simulink model "FOCCONTROL"  (R2022a)
settings: Solver=ode1  StartTime=0.0  StopTime=10  FixedStep=1e-5  RelTol=1e-5  AbsTol=1e-5
values from neighbouring files (symbols this model uses):
  A = [0 -Lq  ; Ld 0 ]    [PMSMParameters.m]
  C0 = 3.53*10.^-1    (= 0.353)    [PMSMParameters.m]
  F = 1.57*10.^-3    (= 0.00157)    [PMSMParameters.m]
  J = 5.21*10.^-3    (= 0.00521)    [PMSMParameters.m]
  Kid = Ld*((wne).^2)/Kpd    [PMSMParameters.m]
  Kim = J*((wnm).^2)/Kpm    [PMSMParameters.m]
  Kiq = Lq*((wne).^2)/Kpq    [PMSMParameters.m]
  Kpd = 2*wne*Ld*ceff-Rs    (= 1472.1)    [PMSMParameters.m]
  Kpm = 2*wnm*J*ceff-F    (= 0.25893)    [PMSMParameters.m]
  Kpq = 2*wne*Lq*ceff-Rs    (= 1122.1)    [PMSMParameters.m]
  L = [Ld 0 ; 0 Lq ]    [PMSMParameters.m]
  Ld = 0.3    [PMSMParameters.m]
  Lq = 0.23    [PMSMParameters.m]
  P = 2    [PMSMParameters.m]
  pf = 1.12    [PMSMParameters.m]
  phif = [0 ; pf]    [PMSMParameters.m]
  R = [Rs 0; 0 Rs ]    [PMSMParameters.m]
  Td = 1/fd    (= 0.001)    [PMSMParameters.m]
  VDC = 600    [PMSMParameters.m]
  VP = VDC    (= 600)    [PMSMParameters.m]
libraries: simulink x1
settings Model: Creator=ZinouAb  LastModifiedBy=ZinouAb
settings ModelReferenceCC: EnableRefExpFcnMdlSchedulingChecks=off
settings RTWCC: Description=Generic Real-Time Target

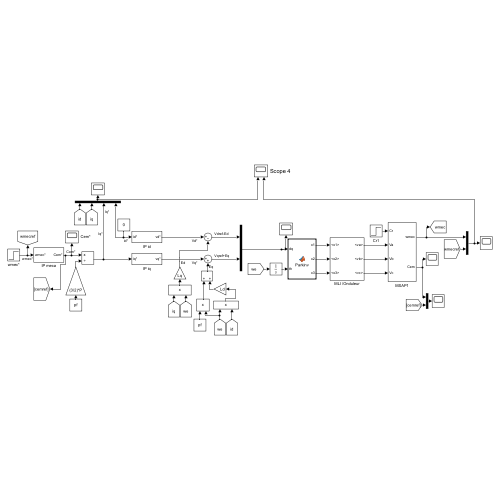
[thumbnail: Simulink's stored preview of the top-level diagram]
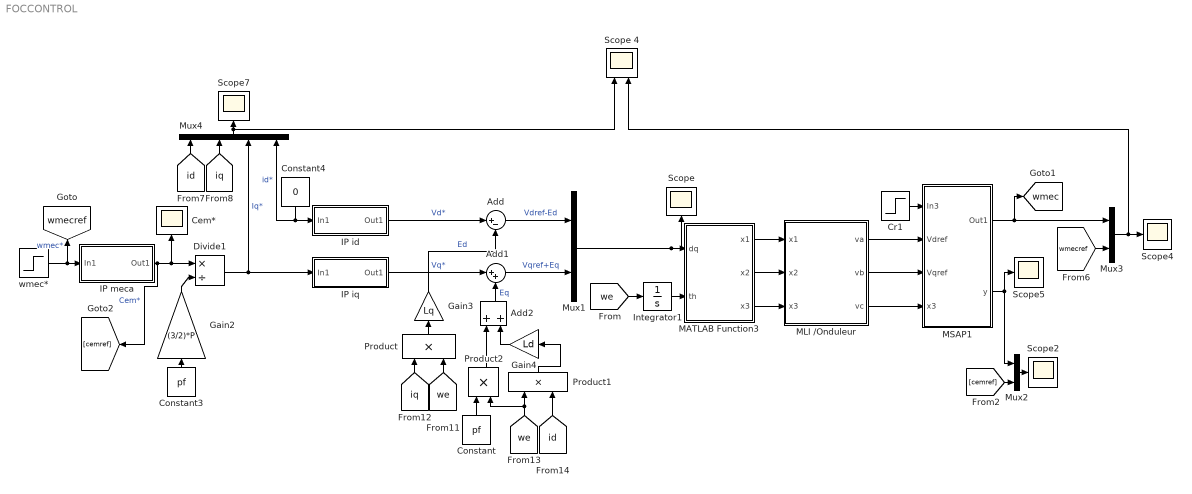
== system FOCCONTROL ==
  Add : Sum  Inputs=|+-
  Add1 : Sum  Inputs=|++
  Add2 : Sum
  Cem* : Scope
  Constant : Constant  Value=pf
  Constant3 : Constant  Value=pf
  Constant4 : Constant  Value=0
  Cr1 : Step  Time=6  After=1.9+C0  SampleTime=0
  Divide1 : Product  Inputs=*/
  Gain2 : Gain  Gain=(3/2)*P
  Gain3 : Gain  Gain=Lq
  Gain4 : Gain  Gain=Ld
  IP id : Subsystem
  IP iq : Subsystem
  IP meca : Subsystem
  Integrator1 : Integrator
  MATLAB Function3 : MATLAB Function  TreatAsAtomicUnit=on
  MLI /Onduleur : Subsystem
  MSAP1 : Subsystem
  Mux1 : Mux  Inputs=2
  Mux2 : Mux  Inputs=2
  Mux3 : Mux  Inputs=2
  Mux4 : Mux
  Product : Product
  Product1 : Product
  Product2 : Product
  Scope{,2,4..5,7} (5 alike) : Scope
  Scope 4 : Scope  NumInputPorts=2
  wmec* : Step  Time=4  After=157  SampleTime=0
  tag scope: wmec=global, wmecref=global
  wires:
  [we] -> Product/2
  MSAP1/2(y) -> Scope5/1, Mux2/1
  Gain4/1 -> Add2/2
  Constant/1 -> Product2/1
  [we] -> Product2/2, Product1/1
  Product2/1 -> Add2/1
  Product/1 -> Gain3/1
  IP iq/1(Out1) -> Add1/1  "Vq*"
  Add2/1 -> Add1/2  "Eq"
  Gain3/1 -> Add/2  "Ed"
  Product1/1 -> Gain4/1
  [id] -> Product1/2
  [iq] -> Product/1
  Constant3/1 -> Gain2/1
  Mux3/1 -> Scope 4/2, Scope4/1
  IP id/1(Out1) -> Add/1  "Vd*"
  Constant4/1 -> IP id/1(In1), Mux4/4  "id*"
  [wmecref] -> Mux3/2
  [id] -> Mux4/1
  Divide1/1 -> IP iq/1(In1), Mux4/3  "Iq*"
  wmec*/1 -> IP meca/1(In1), [wmecref]  "wmec*"
  IP meca/1(Out1) -> Divide1/1, Cem*/1, [cemref]  "Cem*"
  [iq] -> Mux4/2
  Gain2/1 -> Divide1/2
  Cr1/1 -> MSAP1/1(In3)
  Add1/1 -> Mux1/2  "Vqref+Eq"
  Integrator1/1 -> MATLAB Function3/2(th)
  Add/1 -> Mux1/1  "Vdref-Ed"
  [we] -> Integrator1/1
  Mux1/1 -> Scope/1, MATLAB Function3/1(dq)
  MLI /Onduleur/2(vb) -> MSAP1/3(Vqref)
  MLI /Onduleur/1(va) -> MSAP1/2(Vdref)
  MLI /Onduleur/3(vc) -> MSAP1/4(x3)
  MATLAB Function3/1(x1) -> MLI /Onduleur/1(x1)
  MATLAB Function3/2(x2) -> MLI /Onduleur/2(x2)
  MATLAB Function3/3(x3) -> MLI /Onduleur/3(x3)
  [cemref] -> Mux2/2
  Mux2/1 -> Scope2/1
  MSAP1/1(Out1) -> [wmec], Mux3/1
  Mux4/1 -> Scope 4/1, Scope7/1

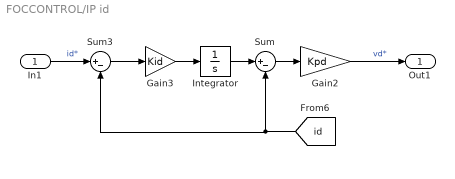
== system FOCCONTROL/IP id ==
  In1 : Inport
  Gain2 : Gain  Gain=Kpd
  Gain3 : Gain  Gain=Kid
  Integrator : Integrator
  Sum : Sum  Inputs=|+-
  Sum3 : Sum  Inputs=|+-
  Out1 : Outport
  wires:
  Integrator/1 -> Sum/1
  [id] -> Sum3/2, Sum/2
  Sum/1 -> Gain2/1
  Gain2/1 -> Out1/1  "vd*"
  Gain3/1 -> Integrator/1
  Sum3/1 -> Gain3/1
  In1/1 -> Sum3/1  "id*"

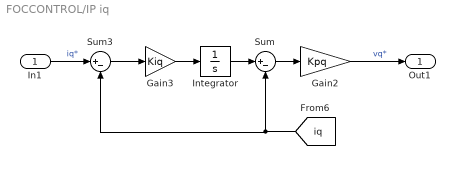
== system FOCCONTROL/IP iq ==
  In1 : Inport
  Gain2 : Gain  Gain=Kpq
  Gain3 : Gain  Gain=Kiq
  Integrator : Integrator
  Sum : Sum  Inputs=|+-
  Sum3 : Sum  Inputs=|+-
  Out1 : Outport
  wires:
  Integrator/1 -> Sum/1
  [iq] -> Sum3/2, Sum/2
  Sum/1 -> Gain2/1
  Gain2/1 -> Out1/1  "vq*"
  Gain3/1 -> Integrator/1
  Sum3/1 -> Gain3/1
  In1/1 -> Sum3/1  "iq*"

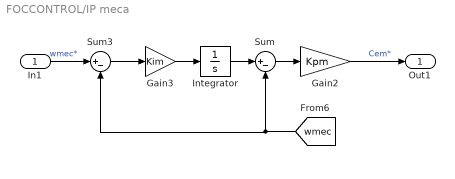
== system FOCCONTROL/IP meca ==
  In1 : Inport
  Gain2 : Gain  Gain=Kpm
  Gain3 : Gain  Gain=Kim
  Integrator : Integrator
  Sum : Sum  Inputs=|+-
  Sum3 : Sum  Inputs=|+-
  Out1 : Outport
  wires:
  Integrator/1 -> Sum/1
  [wmec] -> Sum3/2, Sum/2
  Sum/1 -> Gain2/1
  Gain2/1 -> Out1/1  "Cem*"
  Gain3/1 -> Integrator/1
  Sum3/1 -> Gain3/1
  In1/1 -> Sum3/1  "wmec*"

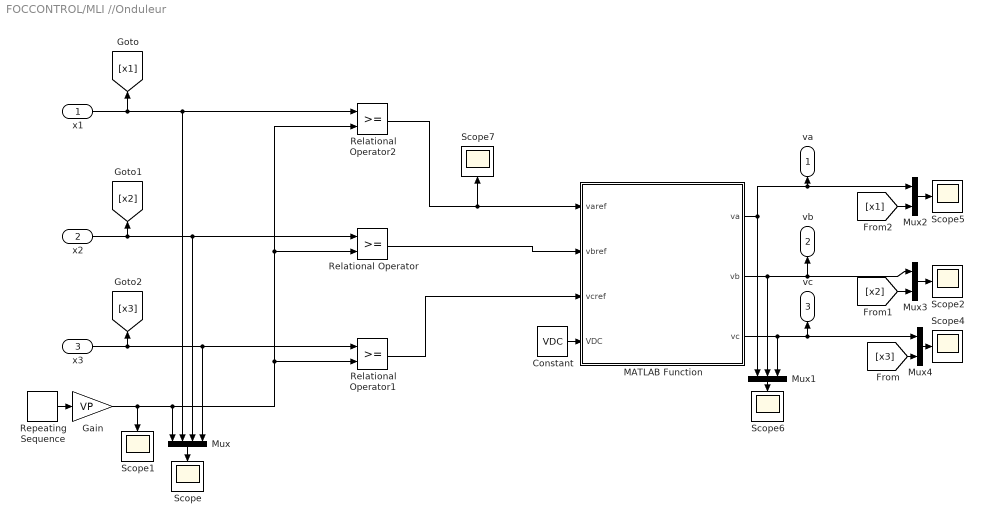
== system FOCCONTROL/MLI //Onduleur ==
  x1 : Inport
  x2 : Inport  Port=2
  x3 : Inport  Port=3
  Constant : Constant  Value=VDC
  Gain : Gain  Gain=VP
  MATLAB Function : MATLAB Function  TreatAsAtomicUnit=on
  Mux : Mux
  Mux1 : Mux  Inputs=3
  Mux2 : Mux  Inputs=2
  Mux3 : Mux  Inputs=2
  Mux4 : Mux  Inputs=2
  Relational Operator : RelationalOperator  OutDataTypeStr=boolean  RndMeth=Simplest  InputSameDT=off
  Relational Operator1 : RelationalOperator  OutDataTypeStr=boolean  RndMeth=Simplest  InputSameDT=off
  Relational Operator2 : RelationalOperator  OutDataTypeStr=boolean  RndMeth=Simplest  InputSameDT=off
  Repeating Sequence : simulink/Sources/Repeating Sequence  rep_seq_t=[0 0.5 1].*Td  rep_seq_y=[-1 1 -1]
  Scope{,1..2,4..7} (7 alike) : Scope
  va : Outport
  vb : Outport  Port=2
  vc : Outport  Port=3
  wires:
  Mux/1 -> Scope/1
  Gain/1 -> Scope1/1, Mux/1, Relational Operator1/2, Relational Operator/2, Relational Operator2/2
  Relational Operator/1 -> MATLAB Function/2(vbref)
  Relational Operator1/1 -> MATLAB Function/3(vcref)
  Relational Operator2/1 -> MATLAB Function/1(varef), Scope7/1
  MATLAB Function/1(va) -> va/1, Mux2/1, Mux1/1
  Constant/1 -> MATLAB Function/4(VDC)
  Mux1/1 -> Scope6/1
  Mux2/1 -> Scope5/1
  MATLAB Function/2(vb) -> Mux1/2, vb/1, Mux3/1
  Mux3/1 -> Scope2/1
  MATLAB Function/3(vc) -> Mux1/3, Mux4/1, vc/1
  Mux4/1 -> Scope4/1
  x1/1 -> [x1], Mux/2, Relational Operator2/1
  x2/1 -> Relational Operator/1, Mux/3, [x2]
  x3/1 -> [x3], Mux/4, Relational Operator1/1
  Repeating Sequence/1 -> Gain/1
  [x2] -> Mux3/2
  [x3] -> Mux4/2
  [x1] -> Mux2/2

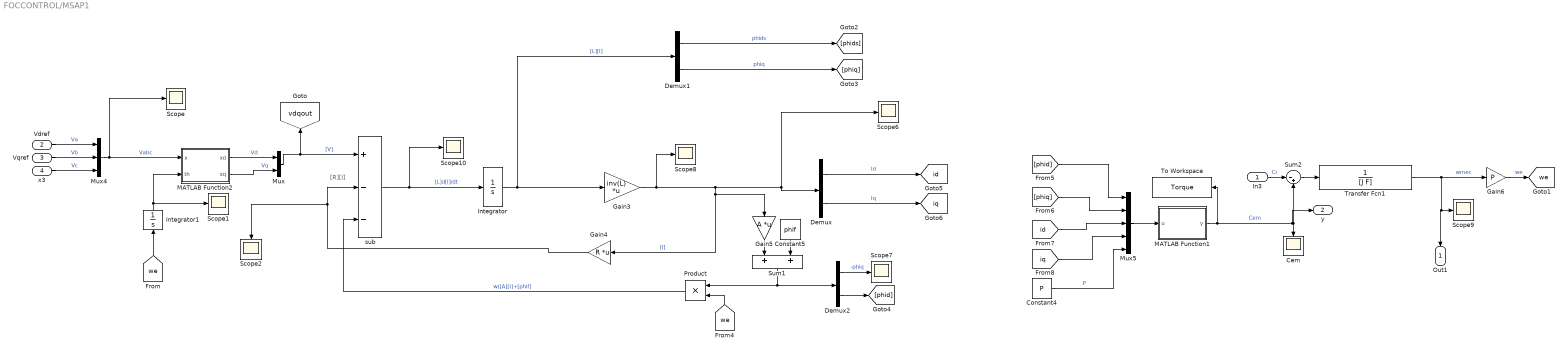
== system FOCCONTROL/MSAP1 ==
  note: [R][I]
  In3 : Inport
  Vdref : Inport  Port=2
  Vqref : Inport  Port=3
  x3 : Inport  Port=4
  Cem : Scope
  Constant4 : Constant  Value=P
  Constant5 : Constant  Value=phif
  Demux : Demux  Outputs=2
  Demux1 : Demux  Outputs=2
  Demux2 : Demux  Outputs=2
  Gain3 : Gain  Gain=inv(L)  Multiplication=Matrix(K*u)
  Gain4 : Gain  Gain=R  Multiplication=Matrix(K*u)
  Gain5 : Gain  Gain=A  Multiplication=Matrix(K*u)
  Gain6 : Gain  Gain=P
  Integrator : Integrator
  Integrator1 : Integrator
  MATLAB Function1 : MATLAB Function  TreatAsAtomicUnit=on
  MATLAB Function2 : MATLAB Function  TreatAsAtomicUnit=on
  Mux : Mux  Inputs=2
  Mux4 : Mux  Inputs=3
  Mux5 : Mux  Inputs=5
  Product : Product
  Scope{,1..2,6..10} (8 alike) : Scope
  Sum1 : Sum
  Sum2 : Sum  Inputs=|-+
  To Workspace : ToWorkspace  VariableName=Torque  SaveFormat=Timeseries  SampleTime=-1
  Transfer Fcn1 : TransferFcn  Denominator=[J F]
  sub : Sum  Inputs=+--
  Out1 : Outport
  y : Outport  Port=2
  tag scope: id=global, iq=global, vdqout=global, we=global
  wires:
  sub/1 -> Scope10/1, Integrator/1  "[L]d[I]/dt"
  MATLAB Function1/1(y) -> Cem/1, Sum2/2, y/1, To Workspace/1  "Cem"
  Product/1 -> sub/3  "w([A][I]+[phif]"
  Sum2/1 -> Transfer Fcn1/1
  Transfer Fcn1/1 -> Out1/1, Scope9/1, Gain6/1  "wmec"
  Vdref/1 -> Mux4/1  "Va"
  Gain4/1 -> Scope2/1, sub/2
  Gain6/1 -> [we]  "we"
  Demux/2 -> [iq]  "Iq"
  Sum1/1 -> Product/1, Demux2/1
  Demux1/2 -> [phiq]  "phiq"
  Integrator/1 -> Gain3/1, Demux1/1  "[L][I]"
  Constant4/1 -> Mux5/5  "P"
  Demux/1 -> [id]  "Id"
  [we] -> Product/2
  Gain5/1 -> Sum1/1
  Gain3/1 -> Gain4/1, Gain5/1, Scope6/1, Demux/1, Scope8/1  "[I]"
  Vqref/1 -> Mux4/2  "Vb"
  Mux5/1 -> MATLAB Function1/1(u)
  In3/1 -> Sum2/1  "Cr"
  Constant5/1 -> Sum1/2
  [id] -> Mux5/3
  [iq] -> Mux5/4
  Demux2/2 -> [phid]
  Demux2/1 -> Scope7/1  "-phiq"
  Mux/1 -> [vdqout], sub/1  "[V]"
  Demux1/1 -> [phids]  "phids"
  [phid] -> Mux5/1
  [phiq] -> Mux5/2
  x3/1 -> Mux4/3  "Vc"
  Mux4/1 -> Scope/1, MATLAB Function2/1(x)  "Vabc"
  MATLAB Function2/1(xd) -> Mux/1  "Vd"
  MATLAB Function2/2(xq) -> Mux/2  "Vq"
  [we] -> Integrator1/1
  Integrator1/1 -> Scope1/1, MATLAB Function2/2(th)

== matlab function FOCCONTROL/MATLAB Function3 ==
  data: dq input; x1 output; x2 output; x3 output; th input
function [x1,x2,x3]= Parkinv(dq,th)
parkinv = [ cos(th),           -sin(th); 
          cos(th-2*pi/3), -sin(th-2*pi/3); 
          cos(th+2*pi/3), -sin(th+2*pi/3)];
temp = parkinv * [dq];
x1=temp(1);
x2=temp(2);
x3=temp(3);

== matlab function FOCCONTROL/MLI //Onduleur/MATLAB Function ==
  data: varef input; vbref input; vcref input; VDC input; va output; vb output; vc output
function [va,vb,vc]= OnduleurOut(varef,vbref,vcref,VDC)
varef=double(varef);
vbref=double(vbref);
vcref=double(vcref);
va=(2*varef-vbref-vcref)*(VDC/3);
vb=(2*vbref-varef-vcref)*(VDC/3);
vc=(2*vcref-vbref-varef)*(VDC/3);

== matlab function FOCCONTROL/MSAP1/MATLAB Function1 ==
  data: u input; y output
function y = CEM(u)

y =(3/2)*u(5)*(u(1)*u(4)-u(2)*u(3));

== matlab function FOCCONTROL/MSAP1/MATLAB Function2 ==
  data: x input; xd output; xq output; th input
function [xd,xq] = Park(x,th)
% vd=(2/3)*(u1*cos(th)+u2*cos(th-2*pi/3)+u3*cos(th+2*pi/3));
% vq=(2/3)*(-u1*sin(th)-u2*sin(th-2*pi/3)-u3*sin(th+2*pi/3));
P=(2/3)*[ cos(th) cos(th-2*pi/3) cos(th+2*pi/3);
         -sin(th) -sin(th-2*pi/3) -sin(th+2*pi/3)  ];
prod=P*x;
xd=prod(1);
xq=prod(2);
